simulink model "Sym_ex5"  (R2021b)
settings: Solver=VariableStepAuto  StartTime=0.0  StopTime=10.0  RelTol=1e-3
libraries: simulink x2
settings Model: Creator=Leonardo  LastModifiedBy=Leonardo

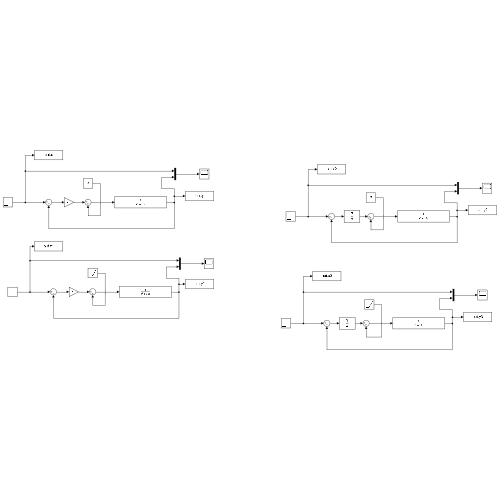
[thumbnail: Simulink's stored preview of the top-level diagram]
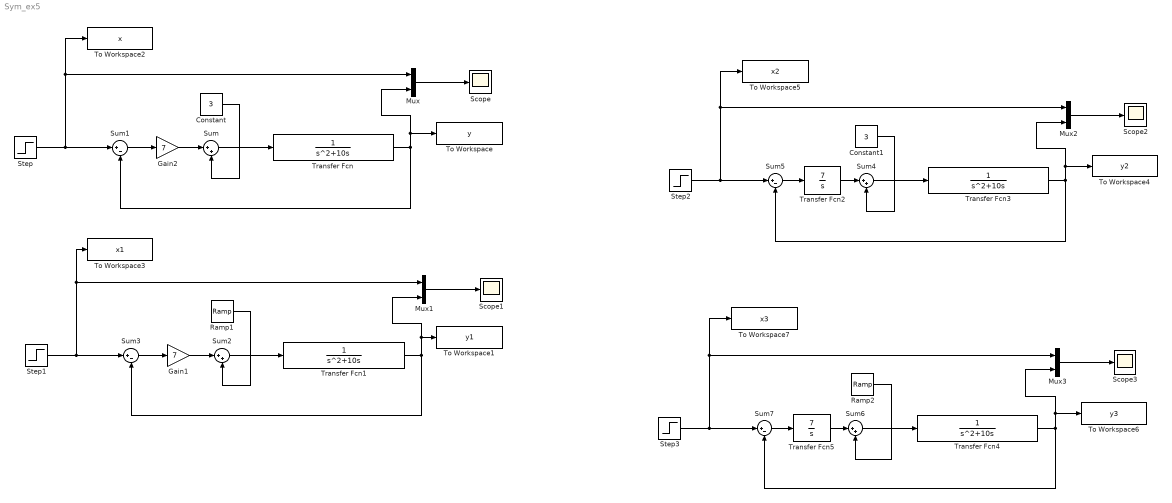
== system Sym_ex5 ==
  Constant : Constant  Value=3
  Constant1 : Constant  Value=3
  Gain1 : Gain  Gain=7
  Gain2 : Gain  Gain=7
  Mux{,1..3} (4 alike) : Mux  Inputs=2
  Ramp1 : simulink/Sources/Ramp  slope=1  start=0  InitialOutput=0
  Ramp2 : simulink/Sources/Ramp  slope=1  start=0  InitialOutput=0
  Scope{,1..3} (4 alike) : Scope
  Step{,1..3} (4 alike) : Step  SampleTime=0
  Sum{,2,4,6} (4 alike) : Sum  Inputs=|++
  Sum{1,3,5,7} (4 alike) : Sum  Inputs=|+-
  To Workspace : ToWorkspace  VariableName=y  SaveFormat=Structure With Time  SampleTime=-1
  To Workspace1 : ToWorkspace  VariableName=y1  SaveFormat=Structure With Time  SampleTime=-1
  To Workspace2 : ToWorkspace  VariableName=x  SaveFormat=Structure With Time  SampleTime=-1
  To Workspace3 : ToWorkspace  VariableName=x1  SaveFormat=Structure With Time  SampleTime=-1
  To Workspace4 : ToWorkspace  VariableName=y2  SaveFormat=Structure With Time  SampleTime=-1
  To Workspace5 : ToWorkspace  VariableName=x2  SaveFormat=Structure With Time  SampleTime=-1
  To Workspace6 : ToWorkspace  VariableName=y3  SaveFormat=Structure With Time  SampleTime=-1
  To Workspace7 : ToWorkspace  VariableName=x3  SaveFormat=Structure With Time  SampleTime=-1
  Transfer Fcn{,1,3..4} (4 alike) : TransferFcn  Denominator=[1 10 0]
  Transfer Fcn2 : TransferFcn  Numerator=[7]  Denominator=[1 0]
  Transfer Fcn5 : TransferFcn  Numerator=[7]  Denominator=[1 0]
  wires:
  Sum5/1 -> Transfer Fcn2/1
  Sum/1 -> Transfer Fcn/1
  Step2/1 -> To Workspace5/1, Mux2/1, Sum5/1
  Ramp2/1 -> Sum6/2
  Step3/1 -> To Workspace7/1, Mux3/1, Sum7/1
  Transfer Fcn5/1 -> Sum6/1
  Constant1/1 -> Sum4/2
  Gain1/1 -> Sum2/1
  Sum7/1 -> Transfer Fcn5/1
  Transfer Fcn4/1 -> To Workspace6/1, Mux3/2, Sum7/2
  Transfer Fcn/1 -> To Workspace/1, Mux/2, Sum1/2
  Mux2/1 -> Scope2/1
  Mux3/1 -> Scope3/1
  Transfer Fcn2/1 -> Sum4/1
  Mux/1 -> Scope/1
  Sum1/1 -> Gain2/1
  Transfer Fcn1/1 -> To Workspace1/1, Mux1/2, Sum3/2
  Gain2/1 -> Sum/1
  Sum3/1 -> Gain1/1
  Step1/1 -> To Workspace3/1, Mux1/1, Sum3/1
  Transfer Fcn3/1 -> To Workspace4/1, Mux2/2, Sum5/2
  Sum6/1 -> Transfer Fcn4/1
  Step/1 -> To Workspace2/1, Mux/1, Sum1/1
  Ramp1/1 -> Sum2/2
  Sum2/1 -> Transfer Fcn1/1
  Mux1/1 -> Scope1/1
  Constant/1 -> Sum/2
  Sum4/1 -> Transfer Fcn3/1
